simulink model "MSMP_CAEHP"  (R2016a)
settings: Solver=ode4  StartTime=0.0  StopTime=1  FixedStep=h  RelTol=1e-3
undefined symbols (not defined in the file): B, J, LambdaPM, Ld, Lq, p, R
settings Model: Creator=student  LastModifiedBy=razva

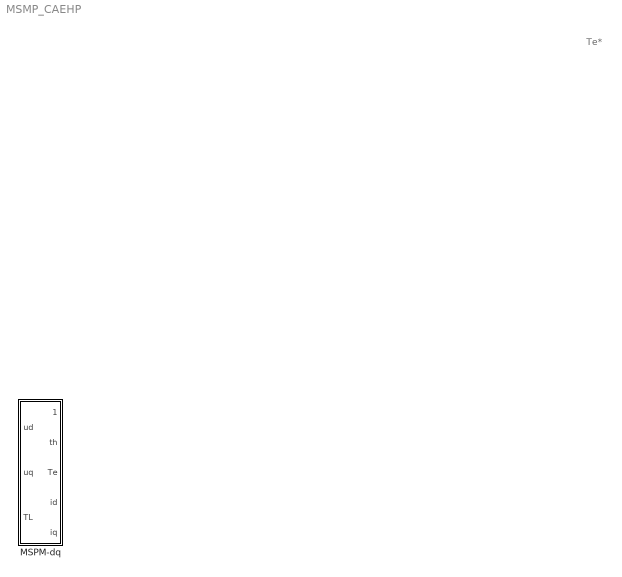
== system MSMP_CAEHP ==
  note: Te*
  MSPM-dq : Subsystem

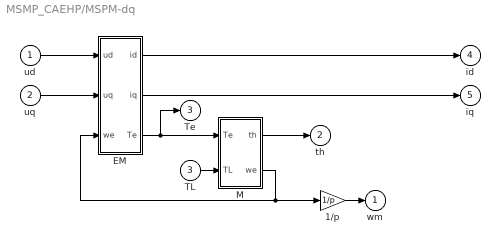
== system MSMP_CAEHP/MSPM-dq ==
  ud : Inport
  uq : Inport  Port=2
  TL : Inport  Port=3
  1/p : Gain  Gain=1/p  SaturateOnIntegerOverflow=on  OutDataTypeStr=Inherit: Same as input  ParamDataTypeStr=Inherit: Same as input
  EM : Subsystem
  M : Subsystem
  wm : Outport  InitialOutput=0
  th : Outport  Port=2  InitialOutput=0
  Te : Outport  Port=3  InitialOutput=0
  id : Outport  Port=4  InitialOutput=0
  iq : Outport  Port=5  InitialOutput=0
  wires:
  M/1(th) -> th/1
  1/p/1 -> wm/1
  ud/1 -> EM/1(ud)
  uq/1 -> EM/2(uq)
  TL/1 -> M/2(TL)
  M/2(we) -> EM/3(we), 1/p/1
  EM/3(Te) -> M/1(Te), Te/1
  EM/1("id ") -> id/1
  EM/2("iq ") -> iq/1

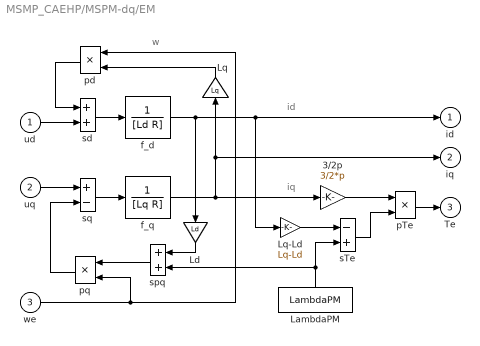
== system MSMP_CAEHP/MSPM-dq/EM ==
  note: w
  note: iq
  note: id
  ud : Inport
  uq : Inport  Port=2
  we : Inport  Port=3
  3/2p : Gain  Gain=3/2*p  SaturateOnIntegerOverflow=on  OutDataTypeStr=Inherit: Same as input  ParamDataTypeStr=Inherit: Same as input
  "LambdaPM " : Constant  Value=LambdaPM
  Ld : Gain  Gain=Ld  SaturateOnIntegerOverflow=on  OutDataTypeStr=Inherit: Same as input  ParamDataTypeStr=Inherit: Same as input
  Lq : Gain  Gain=Lq  SaturateOnIntegerOverflow=on  OutDataTypeStr=Inherit: Same as input  ParamDataTypeStr=Inherit: Same as input
  Lq-Ld : Gain  Gain=Lq-Ld  SaturateOnIntegerOverflow=on  OutDataTypeStr=Inherit: Same as input  ParamDataTypeStr=Inherit: Same as input
  f_d : TransferFcn  Denominator=[Ld R]
  f_q : TransferFcn  Denominator=[Lq R]
  pTe : Product  SaturateOnIntegerOverflow=on  RndMeth=Zero  InputSameDT=on  OutDataTypeStr=Inherit: Same as first input
  pd : Product  SaturateOnIntegerOverflow=on  RndMeth=Zero  InputSameDT=on  OutDataTypeStr=Inherit: Same as first input
  pq : Product  SaturateOnIntegerOverflow=on  RndMeth=Zero  InputSameDT=on  OutDataTypeStr=Inherit: Same as first input
  sTe : Sum  Inputs=-+  SaturateOnIntegerOverflow=on  InputSameDT=on  OutDataTypeStr=Inherit: Same as first input
  sd : Sum  SaturateOnIntegerOverflow=on  InputSameDT=on  OutDataTypeStr=Inherit: Same as first input
  spq : Sum  SaturateOnIntegerOverflow=on  InputSameDT=on  OutDataTypeStr=Inherit: Same as first input
  sq : Sum  Inputs=+-  SaturateOnIntegerOverflow=on  InputSameDT=on  OutDataTypeStr=Inherit: Same as first input
  "id " : Outport  InitialOutput=0
  "iq " : Outport  Port=2  InitialOutput=0
  Te : Outport  Port=3  InitialOutput=0
  wires:
  ud/1 -> sd/2
  uq/1 -> sq/1
  f_d/1 -> Ld/1, Lq-Ld/1, "id "/1
  "LambdaPM "/1 -> spq/2, sTe/2
  f_q/1 -> "iq "/1, Lq/1, 3/2p/1
  Lq-Ld/1 -> sTe/1
  sTe/1 -> pTe/2
  pTe/1 -> Te/1
  3/2p/1 -> pTe/1
  we/1 -> pq/2, pd/1
  pq/1 -> sq/2
  spq/1 -> pq/1
  Ld/1 -> spq/1
  Lq/1 -> pd/2
  pd/1 -> sd/1
  sq/1 -> f_q/1
  sd/1 -> f_d/1

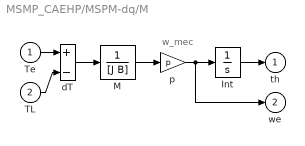
== system MSMP_CAEHP/MSPM-dq/M ==
  note: w_mec
  Te : Inport
  TL : Inport  Port=2
  Int : Integrator
  M : TransferFcn  Denominator=[J B]
  dT : Sum  Inputs=+-  SaturateOnIntegerOverflow=on  InputSameDT=on  OutDataTypeStr=Inherit: Same as first input
  p : Gain  Gain=p  SaturateOnIntegerOverflow=on  OutDataTypeStr=Inherit: Same as input  ParamDataTypeStr=Inherit: Same as input
  th : Outport  InitialOutput=0
  we : Outport  Port=2  InitialOutput=0
  wires:
  dT/1 -> M/1
  M/1 -> p/1
  TL/1 -> dT/2
  p/1 -> Int/1, we/1
  Int/1 -> th/1
  Te/1 -> dT/1
